simulink model "dynamic_calib"  (Simulink 8.8)
settings: Solver=FixedStepDiscrete  StartTime=0.0  StopTime=tEnd  FixedStep=CONFIG.Ts  RelTol=1e-3  EnableMultiTasking=on
undefined symbols (not defined in the file or in its folder): calibDelta, tSwitch, USE_h_ONLY
libraries: WBToolboxLibrary x18
settings Model: SuppressorTable=22 serialization::archive 11 0 3 0 0 0 11 0  Creator=gabri  LastModifiedBy=gnava
settings DataIOCC: SignalLoggingSaveFormat=Dataset
settings DebuggingCC: UnderspecifiedInitializationDetection=Simplified  MergeDetectMultiDrivingBlocksExec=error  SolverPrmCheckMsg=warning  FcnCallInpInsideContextMsg=error  StateNameClashWarn=none
settings GRTTargetCC: CombineOutputUpdateFcns=on  GRTInterface=off
settings ConfigComp: CovSFcnEnable=off

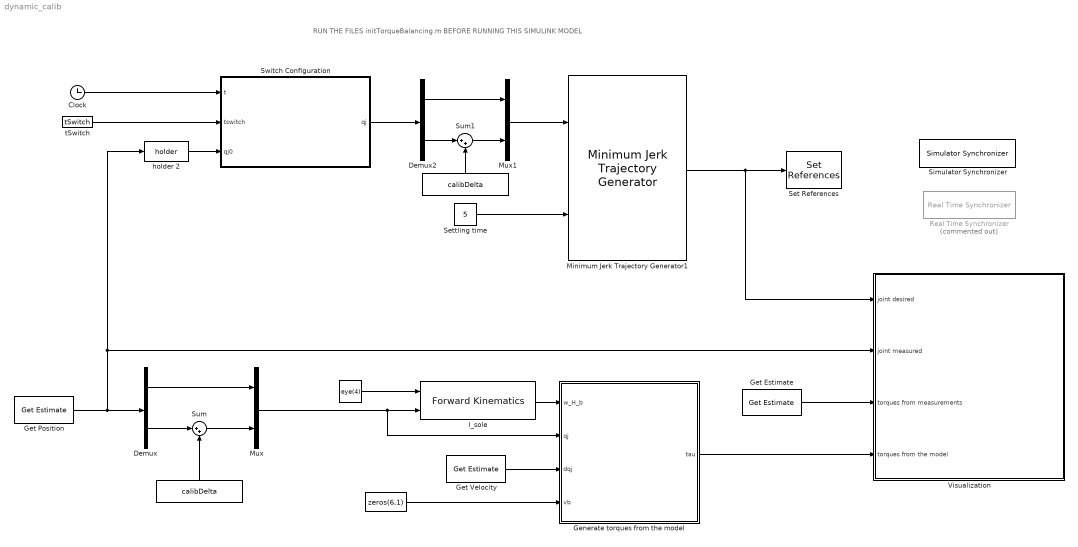
== system dynamic_calib ==
  note: RUN THE FILES initTorqueBalancing.m BEFORE RUNNING THIS SIMULINK MODEL
  " " : Constant  Value=eye(4)
  "           " : Constant  Value=zeros(6,1)
  "                   " : Constant  Value=calibDelta
  "                                                      " : Constant  Value=calibDelta
  Clock : Clock
  Demux : Demux  Outputs=[13;12]
  Demux2 : Demux  Outputs=[13;12]
  Generate torques from the model : Subsystem
  Get Estimate : WBToolboxLibrary/wholeBodyStates/Get Estimate  estimateType=Joints Torque  robotName=WBT_robotName  localName=WBT_modelName  wbiFile=WBT_wbiFilename  wbiList=WBT_wbiList
  Get Position : WBToolboxLibrary/wholeBodyStates/Get Estimate  estimateType=Joints Position  robotName=WBT_robotName  localName=WBT_modelName  wbiFile=WBT_wbiFilename  wbiList=WBT_wbiList
  Get Velocity : WBToolboxLibrary/wholeBodyStates/Get Estimate  estimateType=Joints Velocity  robotName=WBT_robotName  localName=WBT_modelName  wbiFile=WBT_wbiFilename  wbiList=WBT_wbiList
  Minimum Jerk Trajectory Generator1 : WBToolboxLibrary/Utilities/Minimum Jerk Trajectory Generator  externalSettlingTime=on  settlingTime=1  sampleTime=CONFIG.Ts  resetOnSettlingTime=off  firstDerivatives=off  secondDerivatives=off  explicitInitialValue=off
  Mux : Mux  Inputs=2
  Mux1 : Mux  Inputs=2
  Real Time Synchronizer : WBToolboxLibrary/Utilities/Real Time Synchronizer  Commented=on  period=0.01
  Set References : WBToolboxLibrary/wholeBodyActuators/Set References  controlType=Position Direct  fullOrSubControl=Full  controlledJoints=''  robotName=WBT_robotName  localName=WBT_modelName  wbiFile=WBT_wbiFilename  wbiList=WBT_wbiList
  Settling time : Constant  Value=5
  Simulator Synchronizer : WBToolboxLibrary/Utilities/Simulator Synchronizer  period=0.01  serverPortName='/clock/rpc'  clientPortName='/WBT_synchronizer/rpc:o'
  Sum : Sum  Inputs=|++
  Sum1 : Sum  Inputs=|++
  Switch Configuration : MATLAB Function  TreatAsAtomicUnit=on
  Visualization : Subsystem
  holder 2 : WBToolboxLibrary/Utilities/holder 
  l_sole : WBToolboxLibrary/wholeBodyModel/Kinematics/Forward Kinematics  frameName='Waist'  robotName=WBT_robotName  localName=WBT_modelName  wbiFile=WBT_wbiFilename  wbiList=WBT_wbiList
  tSwitch : Constant  Value=tSwitch
  wires:
  "                                                      "/1 -> Sum/2
  Get Estimate/1 -> Visualization/3(torques from measurements)
  Get Position/1 -> holder 2/1, Visualization/2("joint measured "), Demux/1
  Demux/2 -> Sum/1
  Demux/1 -> Mux/1
  Mux/1 -> Generate torques from the model/2(qj), l_sole/2
  Sum/1 -> Mux/2
  Settling time/1 -> Minimum Jerk Trajectory Generator1/2
  Clock/1 -> Switch Configuration/1(t)
  tSwitch/1 -> Switch Configuration/2(tswitch)
  " "/1 -> l_sole/1
  holder 2/1 -> Switch Configuration/3(qj0)
  l_sole/1 -> Generate torques from the model/1(w_H_b)
  Get Velocity/1 -> Generate torques from the model/3(dqj)
  "           "/1 -> Generate torques from the model/4(vb)
  Generate torques from the model/1(tau) -> Visualization/4(torques from the model)
  "                   "/1 -> Sum1/2
  Switch Configuration/1(qj) -> Demux2/1
  Demux2/2 -> Sum1/1
  Demux2/1 -> Mux1/1
  Sum1/1 -> Mux1/2
  Mux1/1 -> Minimum Jerk Trajectory Generator1/1
  Minimum Jerk Trajectory Generator1/1 -> Visualization/1(joint desired), Set References/1

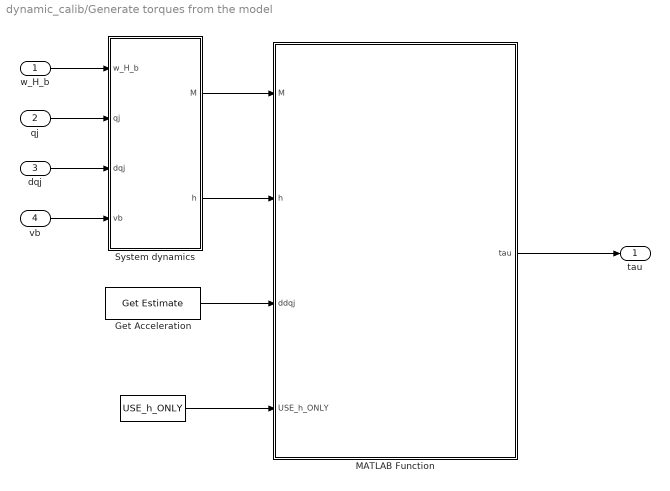
== system dynamic_calib/Generate torques from the model ==
  w_H_b : Inport
  qj : Inport  Port=2
  dqj : Inport  Port=3
  vb : Inport  Port=4
  "           " : Constant  Value=USE_h_ONLY
  Get Acceleration : WBToolboxLibrary/wholeBodyStates/Get Estimate  estimateType=Joints Acceleration  robotName=WBT_robotName  localName=WBT_modelName  wbiFile=WBT_wbiFilename  wbiList=WBT_wbiList
  MATLAB Function : MATLAB Function  TreatAsAtomicUnit=on
  System dynamics : Subsystem
  tau : Outport
  wires:
  qj/1 -> System dynamics/2(qj)
  w_H_b/1 -> System dynamics/1(w_H_b)
  MATLAB Function/1(tau) -> tau/1
  dqj/1 -> System dynamics/3(dqj)
  vb/1 -> System dynamics/4(vb)
  System dynamics/1("M ") -> MATLAB Function/1(M)
  System dynamics/2(h) -> MATLAB Function/2(h)
  Get Acceleration/1 -> MATLAB Function/3(ddqj)
  "           "/1 -> MATLAB Function/4(USE_h_ONLY)

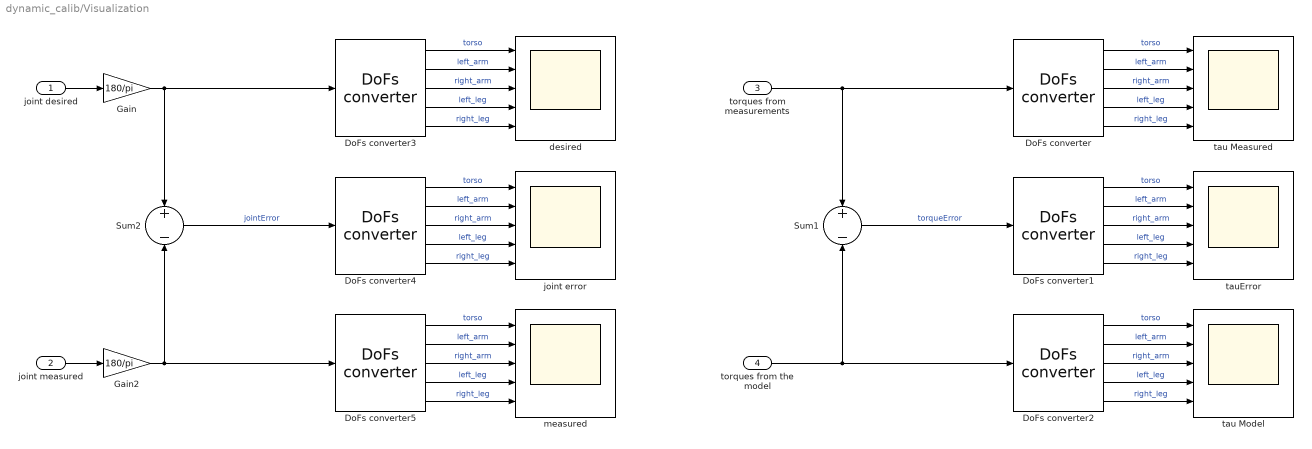
== system dynamic_calib/Visualization ==
  joint desired : Inport
  "joint measured " : Inport  Port=2
  torques from measurements : Inport  Port=3
  torques from the model : Inport  Port=4
  DoFs converter{,1..5} (6 alike) : WBToolboxLibrary/Utilities/DoFs converter  yarp2WBIOption=From WBI to YARP  robotName=WBT_robotName  localName=WBT_modelName  wbiFile=WBT_wbiFilename  wbiList=WBT_wbiList
  Gain : Gain  Gain=180/pi
  Gain2 : Gain  Gain=180/pi
  Sum1 : Sum  Inputs=+-
  Sum2 : Sum  Inputs=+-
  desired : Scope  NumInputPorts=5
  joint error : Scope  NumInputPorts=5
  measured : Scope  NumInputPorts=5
  tau Measured : Scope  NumInputPorts=5
  tau Model : Scope  NumInputPorts=5
  tauError : Scope  NumInputPorts=5
  wires:
  DoFs converter2/3 -> tau Model/3  "right_arm"
  torques from the model/1 -> DoFs converter2/1, Sum1/2
  DoFs converter/4 -> tau Measured/4  "left_leg"
  DoFs converter/3 -> tau Measured/3  "right_arm"
  DoFs converter1/5 -> tauError/5  "right_leg"
  DoFs converter1/1 -> tauError/1  "torso"
  DoFs converter1/2 -> tauError/2  "left_arm"
  DoFs converter1/4 -> tauError/4  "left_leg"
  DoFs converter1/3 -> tauError/3  "right_arm"
  Sum1/1 -> DoFs converter1/1  "torqueError"
  DoFs converter2/5 -> tau Model/5  "right_leg"
  DoFs converter2/1 -> tau Model/1  "torso"
  DoFs converter2/2 -> tau Model/2  "left_arm"
  DoFs converter2/4 -> tau Model/4  "left_leg"
  torques from measurements/1 -> DoFs converter/1, Sum1/1
  DoFs converter/5 -> tau Measured/5  "right_leg"
  DoFs converter/1 -> tau Measured/1  "torso"
  DoFs converter/2 -> tau Measured/2  "left_arm"
  DoFs converter5/3 -> measured/3  "right_arm"
  "joint measured "/1 -> Gain2/1
  DoFs converter3/4 -> desired/4  "left_leg"
  DoFs converter3/3 -> desired/3  "right_arm"
  DoFs converter4/5 -> joint error/5  "right_leg"
  DoFs converter4/1 -> joint error/1  "torso"
  DoFs converter4/2 -> joint error/2  "left_arm"
  DoFs converter4/4 -> joint error/4  "left_leg"
  DoFs converter4/3 -> joint error/3  "right_arm"
  Sum2/1 -> DoFs converter4/1  "jointError"
  DoFs converter5/5 -> measured/5  "right_leg"
  DoFs converter5/1 -> measured/1  "torso"
  DoFs converter5/2 -> measured/2  "left_arm"
  DoFs converter5/4 -> measured/4  "left_leg"
  joint desired/1 -> Gain/1
  DoFs converter3/5 -> desired/5  "right_leg"
  DoFs converter3/1 -> desired/1  "torso"
  DoFs converter3/2 -> desired/2  "left_arm"
  Gain/1 -> DoFs converter3/1, Sum2/1
  Gain2/1 -> DoFs converter5/1, Sum2/2

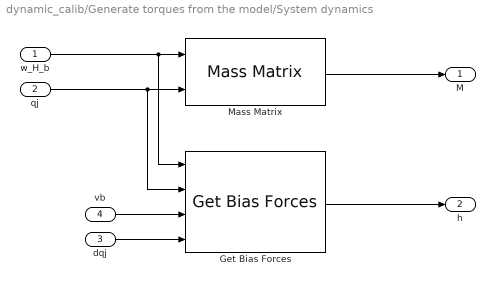
== system dynamic_calib/Generate torques from the model/System dynamics ==
  w_H_b : Inport
  qj : Inport  Port=2
  dqj : Inport  Port=3
  vb : Inport  Port=4
  Get Bias Forces : WBToolboxLibrary/wholeBodyModel/Dynamics/Get Bias Forces  robotName=WBT_robotName  localName=WBT_modelName  wbiFile=WBT_wbiFilename  wbiList=WBT_wbiList  explicitGravity=off
  Mass Matrix : WBToolboxLibrary/wholeBodyModel/Dynamics/Mass Matrix  robotName=WBT_robotName  localName=WBT_modelName  wbiFile=WBT_wbiFilename  wbiList=WBT_wbiList
  "M " : Outport
  h : Outport  Port=2
  wires:
  Mass Matrix/1 -> "M "/1
  Get Bias Forces/1 -> h/1
  w_H_b/1 -> Get Bias Forces/1, Mass Matrix/1
  qj/1 -> Get Bias Forces/2, Mass Matrix/2
  vb/1 -> Get Bias Forces/3
  dqj/1 -> Get Bias Forces/4

== matlab function Generate torques from the model/MATLAB Function ==
  data: M input double; tau output double; h input double; ddqj input double; USE_h_ONLY input double
function tau = computeForwardDynamicsFCN(M,h,ddqj,USE_h_ONLY)

    tau = computeForwardDynamics(M,h,ddqj,USE_h_ONLY);

end

== matlab function Switch Configuration ==
  data: t input double; qj output double; tswitch input double; qj0 input double
function qj = changeConfigFCN(t,tswitch,qj0)

qj = changeConfig(t,tswitch,qj0);

end
